simulink model "Exercise3Simulink"  (R2020a)
settings: Solver=VariableStepAuto  StartTime=0.0  StopTime=1.5  RelTol=1e-3
PreLoadFcn:
  | System.mlx
values from neighbouring files (symbols this model uses):
  A = [0 1 0 0 ... (first row only)    [Exercise3.m]
  B = [0 0 ... (first row only)    [Exercise3.m]
  C = [B A*B A*A*B A*A*A*B]    [Exercise3.m]
undefined symbols (not defined in the file or in its folder): F, Fi, L, M, reference
settings Model: Creator=Emil  LastModifiedBy=Emil

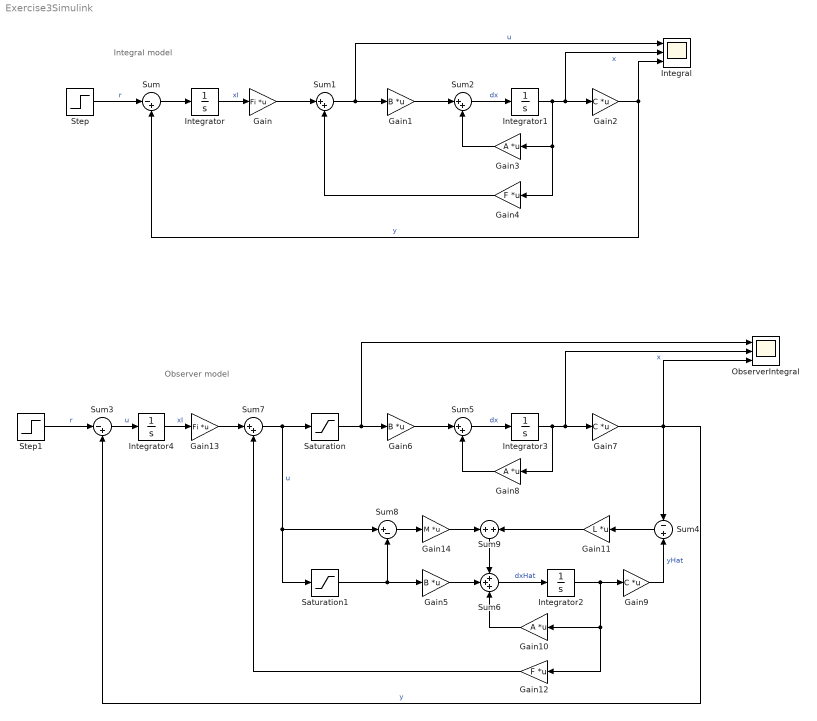
== system Exercise3Simulink ==
  note: Integral model
  note: Observer model
  Gain : Gain  Gain=Fi  Multiplication=Matrix(K*u)
  Gain1 : Gain  Gain=B  Multiplication=Matrix(K*u)
  Gain10 : Gain  Gain=A  Multiplication=Matrix(K*u)
  Gain11 : Gain  Gain=L  Multiplication=Matrix(K*u)
  Gain12 : Gain  Gain=F  Multiplication=Matrix(K*u)
  Gain13 : Gain  Gain=Fi  Multiplication=Matrix(K*u)
  Gain14 : Gain  Gain=M  Multiplication=Matrix(K*u)
  Gain2 : Gain  Gain=C  Multiplication=Matrix(K*u)
  Gain3 : Gain  Gain=A  Multiplication=Matrix(K*u)
  Gain4 : Gain  Gain=F  Multiplication=Matrix(K*u)
  Gain5 : Gain  Gain=B  Multiplication=Matrix(K*u)
  Gain6 : Gain  Gain=B  Multiplication=Matrix(K*u)
  Gain7 : Gain  Gain=C  Multiplication=Matrix(K*u)
  Gain8 : Gain  Gain=A  Multiplication=Matrix(K*u)
  Gain9 : Gain  Gain=C  Multiplication=Matrix(K*u)
  Integral : Scope  NumInputPorts=3
  Integrator{,1..4} (5 alike) : Integrator
  ObserverIntegral : Scope  NumInputPorts=3
  Saturation : Saturate  UpperLimit=40  LowerLimit=-40
  Saturation1 : Saturate  UpperLimit=40  LowerLimit=-40
  Step : Step  Time=0  After=reference  SampleTime=0
  Step1 : Step  Time=0  After=reference  SampleTime=0
  Sum : Sum  Inputs=|-+
  Sum{1..2,5,7} (4 alike) : Sum  Inputs=|++
  Sum3 : Sum  Inputs=|-+
  Sum4 : Sum  Inputs=-+
  Sum6 : Sum  Inputs=+++
  Sum8 : Sum  Inputs=|+-
  Sum9 : Sum
  wires:
  Step/1 -> Sum/1  "r"
  Sum/1 -> Integrator/1
  Integrator/1 -> Gain/1  "xI"
  Gain/1 -> Sum1/1
  Sum1/1 -> Integral/1, Gain1/1  "u"
  Gain1/1 -> Sum2/1
  Sum2/1 -> Integrator1/1  "dx"
  Integrator1/1 -> Gain4/1, Gain3/1, Integral/2, Gain2/1  "x"
  Gain3/1 -> Sum2/2
  Gain4/1 -> Sum1/2
  Gain2/1 -> Integral/3, Sum/2  "y"
  Gain7/1 -> Sum4/1, Sum3/2, ObserverIntegral/3  "y"
  Gain8/1 -> Sum5/2
  Sum5/1 -> Integrator3/1  "dx"
  Gain6/1 -> Sum5/1
  Integrator3/1 -> Gain8/1, ObserverIntegral/2, Gain7/1  "x"
  Gain5/1 -> Sum6/2
  Sum6/1 -> Integrator2/1  "dxHat"
  Integrator2/1 -> Gain10/1, Gain12/1, Gain9/1
  Gain9/1 -> Sum4/2  "yHat"
  Gain10/1 -> Sum6/3
  Sum4/1 -> Gain11/1
  Integrator4/1 -> Gain13/1  "xI"
  Step1/1 -> Sum3/1  "r"
  Sum7/1 -> Sum8/1, Saturation1/1, Saturation/1  "u"
  Sum3/1 -> Integrator4/1  "u"
  Gain13/1 -> Sum7/1
  Gain12/1 -> Sum7/2
  Sum8/1 -> Gain14/1
  Sum9/1 -> Sum6/1
  Gain11/1 -> Sum9/2
  Saturation/1 -> ObserverIntegral/1, Gain6/1
  Saturation1/1 -> Sum8/2, Gain5/1
  Gain14/1 -> Sum9/1
